simulink model "Assignment_2_Group23"  (R2022a)
settings: Solver=FixedStepAuto  StartTime=0.0  StopTime=60  FixedStep=1e-3  RelTol=1e-3  EnableMultiTasking=on
undefined symbols (not defined in the file): D0, D1, D10, D11, D12, D13, D2, D3, D4, D5, D6, D7, D8, D9, PTA0, PTA1, PTA2, PTB23, PTB9, PTC16, PTC17, PTC2, PTC3, PTC4, PTD0, PTD1, PTD2, PTD3
libraries: frdmk64flib x16, etargetslib x1
(part 3 of 3)

== stateflow chart Assignment_2_Group23/Collect//Set Input Parameters ==
  state Input_Parameters
    entry:
    Mode = typecast(RxData(2:3),'uint16')
    LRL = typecast(RxData(4:5),'uint16')
    URL = typecast(RxData(6:7),'uint16')
    Vent_Pulse_W = typecast(RxData(8:9),'uint16')
    Atr_Pulse_W =  typecast(RxData(10:11),'uint16')
    Pulse_Amp = typecast(RxData(12:15),'single');
    Vent_Ref_Period = typecast(RxData(16:17),'uint16');
    Atr_Ref_Period = typecast(RxData(18:19),'uint16');
  state Wait_For_Transmission
  state ECHO_PARAM
    entry:
    send_params();
  Input_Parameters -> Wait_For_Transmission
  (default) -> Wait_For_Transmission
  (junction 63) -> Input_Parameters [order 1] : [RxData(20) == hex2dec('30')]
  (junction 16) -> Wait_For_Transmission [order 2]
  Wait_For_Transmission -> (junction 16) : [Status == 0]
  (junction 16) -> (junction 63) [order 1] : [RxData(1) == hex2dec('10')]
  (junction 63) -> ECHO_PARAM [order 2] : [RxData(20) == hex2dec('32')]
  ECHO_PARAM -> Wait_For_Transmission
  data: RxData input uint8; Status input uint8; Mode output uint16; Atr_Pulse_W output uint16; Atr_Ref_Period output uint16; URL output uint16; Pulse_Amp output single; Vent_Pulse_W output uint16; Vent_Ref_Period output uint16; LRL output uint16

== stateflow chart Assignment_2_Group23/Pacing ==
  state AAI_Refractory_Period
    entry:
    Front_End_Ctrl = false;
    Atr_Gnd_Ctrl = true;
    Atr_Pace_Ctrl = false;
    Pace_Charge_Ctrl = true;
    Front_End_Ctrl = true;
    Sensing_Pace_Cycle = LRL_time - ARP - Atr_Pulse_W;
  state AAI_Charge
    entry:
    Atr_Gnd_Ctrl = true;
    Atr_Pace_Ctrl = false;
    Vent_Pace_Ctrl = false;
    Vent_Gnd_Ctrl = false;
    Pace_Charge_Ctrl = true;
    Sensing_Pace_Cycle = LRL_time - ARP - Atr_Pulse_W;
    Front_End_Ctrl = true;
  state AAI_Pace
    entry:
    Atr_Gnd_Ctrl = false;
    Atr_Pace_Ctrl = true;
    Pace_Charge_Ctrl = false;
  state Initial_State
  state VOO_Charge
    entry:
    Vent_Pace_Ctrl = false;
    Vent_Gnd_Ctrl = true;
    Atr_Gnd_Ctrl = false;
    Atr_Pace_Ctrl = false;
    Front_End_Ctrl = false;
    Pace_Charge_Ctrl = true;
  state VOO_Discharge
    entry:
    Vent_Pace_Ctrl = true;
    Vent_Gnd_Ctrl = false;
    Pace_Charge_Ctrl = false;
  state AOO_Charge
    entry:
    Atr_Gnd_Ctrl = true;
    Atr_Pace_Ctrl = false;
    Vent_Pace_Ctrl = false;
    Vent_Gnd_Ctrl = false;
    Front_End_Ctrl = false;
    Pace_Charge_Ctrl = true;
  state AOO_Discharge
    entry:
    Atr_Gnd_Ctrl = false;
    Atr_Pace_Ctrl = true;
    Pace_Charge_Ctrl = false;
  state VVI_Charge
    entry:
    Vent_Gnd_Ctrl = true;
    Vent_Pace_Ctrl = false;
    Atr_Gnd_Ctrl = false;
    Atr_Pace_Ctrl = false;
    Pace_Charge_Ctrl = true;
    Sensing_Pace_Cycle = LRL_time - VRP - Vent_Pulse_W;
    Front_End_Ctrl = true;
  state VVI_Pace
    entry:
    Vent_Gnd_Ctrl = false;
    Vent_Pace_Ctrl = true;
    Pace_Charge_Ctrl = false;
  state VVI_Refractory_Period
    entry:
    Front_End_Ctrl = false;
    Vent_Gnd_Ctrl = true;
    Vent_Pace_Ctrl = false;
    Pace_Charge_Ctrl = true;
    Front_End_Ctrl = true;
    Sensing_Pace_Cycle = LRL_time - VRP - Vent_Pulse_W;
  AAI_Charge -> AAI_Refractory_Period [order 1] : [Atr_Cmp_Detect == true]{Sensing_Pace_Cycle = LRL_time - ARP}
  AAI_Refractory_Period -> AAI_Charge : after(ARP,msec)
  AAI_Pace -> AAI_Refractory_Period : after(Atr_Pulse_W,msec)
  AAI_Charge -> Initial_State [order 2] : [Mode ~= 4]
  Initial_State -> AAI_Charge [order 2] : [Mode == 4]
  AAI_Charge -> AAI_Pace [order 3] : after(Sensing_Pace_Cycle,msec)
  (default) -> Initial_State
  Initial_State -> VOO_Charge [order 1] : [Mode == 1]
  VOO_Discharge -> VOO_Charge : after(Vent_Pulse_W,msec)
  VOO_Charge -> Initial_State [order 1] : [Mode ~= 1]
  VOO_Charge -> VOO_Discharge [order 2] : [after((LRL_time)-Vent_Pulse_W,msec)]
  AOO_Charge -> Initial_State [order 1] : [Mode ~= 2]
  AOO_Discharge -> AOO_Charge : after(Atr_Pulse_W,msec)
  Initial_State -> AOO_Charge [order 3] : [Mode == 2]
  AOO_Charge -> AOO_Discharge [order 2] : after(LRL_time-Atr_Pulse_W,msec)
  VVI_Charge -> Initial_State [order 1] : [Mode ~= 3]
  Initial_State -> VVI_Charge [order 4] : [Mode == 3]
  VVI_Charge -> VVI_Pace [order 3] : after(Sensing_Pace_Cycle,msec)
  VVI_Pace -> VVI_Refractory_Period : after(Vent_Pulse_W,msec)
  VVI_Charge -> VVI_Refractory_Period [order 2] : [Vent_Cmp_Detect == true]{Sensing_Pace_Cycle = LRL_time - VRP}
  VVI_Refractory_Period -> VVI_Charge : after(VRP,msec)
  data: Mode input uint16; Atr_Pulse_W input uint16; Vent_Pulse_W input uint16; LRL_time input uint16; URL_time input uint16; ARP input uint16; VRP input uint16; Vent_Pace_Ctrl output boolean; Atr_Gnd_Ctrl output boolean; Atr_Pace_Ctrl output boolean; Pace_Charge_Ctrl output boolean; Vent_Gnd_Ctrl output boolean; Sensing_Pace_Cycle local; Front_End_Ctrl output boolean; Vent_Cmp_Detect input boolean; Atr_Cmp_Detect input
